simulink model "bara_thrust_model"  (R2018a)
settings: Solver=FixedStepAuto  StartTime=0.0  StopTime=sim_data3(end,1)  FixedStep=0.0104  RelTol=1e-3
PreLoadFcn:
  | a = 0.03432;
  | b = 0.3933;
  | c = 0.0056;
model workspace (MAT data in the model file):
  a = 0.00307384410727
  a1 = Simulink.Parameter
  a1.Value = 0.03432
  a1.DataType = 'double'
  a1.Dimensions = [1 1]
  b = 0.991162737935
  b1 = Simulink.Parameter
  b1.Value = 0.3933
  b1.DataType = 'auto'
  b1.Dimensions = [1 1]
  c = 0.0571408330036
  c1 = Simulink.Parameter
  c1.Value = 0.0056
  c1.DataType = 'auto'
  c1.Dimensions = [1 1]
  d = 1.70754777062
  e = 2.1214749593
settings Model: ParameterArgumentNames=a,a1,b,b1,c,c1  OrderedModelArguments=off  Creator=emran  LastModifiedBy=emran

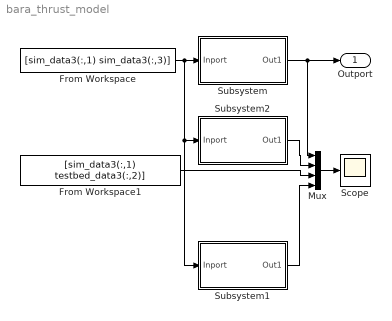
== system bara_thrust_model ==
  From Workspace : FromWorkspace  VariableName=[sim_data3(:,1) sim_data3(:,3)]  SampleTime=0
  From Workspace1 : FromWorkspace  VariableName=[sim_data3(:,1) testbed_data3(:,2)]  SampleTime=0
  Mux : Mux
  Scope : Scope
  Subsystem : Subsystem
  Subsystem1 : Subsystem
  Subsystem2 : Subsystem
  Outport : Outport
  wires:
  From Workspace/1 -> Subsystem2/1(Inport), Subsystem1/1(Inport), Subsystem/1(Inport)
  Subsystem/1(Out1) -> Mux/1, Outport/1
  From Workspace1/1 -> Mux/3
  Mux/1 -> Scope/1
  Subsystem1/1(Out1) -> Mux/4
  Subsystem2/1(Out1) -> Mux/2

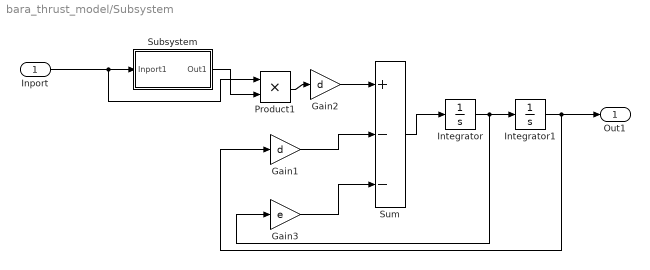
== system bara_thrust_model/Subsystem ==
  Inport : Inport
  Gain1 : Gain  Gain=d
  Gain2 : Gain  Gain=d
  Gain3 : Gain  Gain=e
  Integrator : Integrator
  Integrator1 : Integrator
  Product1 : Product
  Subsystem : Subsystem
  Sum : Sum  Inputs=+--
  Out1 : Outport
  wires:
  Subsystem/1(Out1) -> Product1/2
  Inport/1 -> Product1/1, Subsystem/1(Inport1)
  Integrator/1 -> Gain3/1, Integrator1/1
  Product1/1 -> Gain2/1
  Gain2/1 -> Sum/1
  Integrator1/1 -> Out1/1, Gain1/1
  Sum/1 -> Integrator/1
  Gain3/1 -> Sum/3
  Gain1/1 -> Sum/2

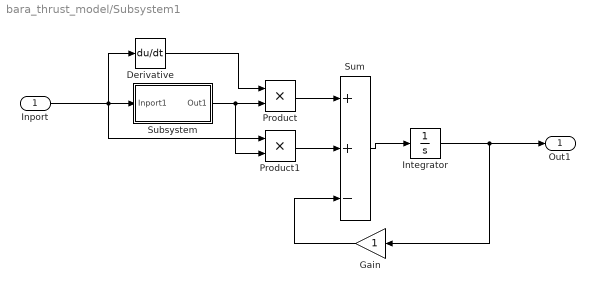
== system bara_thrust_model/Subsystem1 ==
  Inport : Inport
  Derivative : Derivative
  Gain : Gain
  Integrator : Integrator
  Product : Product
  Product1 : Product
  Subsystem : Subsystem
  Sum : Sum  Inputs=++-
  Out1 : Outport
  wires:
  Derivative/1 -> Product/1
  Product1/1 -> Sum/2
  Inport/1 -> Subsystem/1(Inport1), Derivative/1, Product1/1
  Integrator/1 -> Out1/1, Gain/1
  Subsystem/1(Out1) -> Product/2, Product1/2
  Sum/1 -> Integrator/1
  Product/1 -> Sum/1
  Gain/1 -> Sum/3

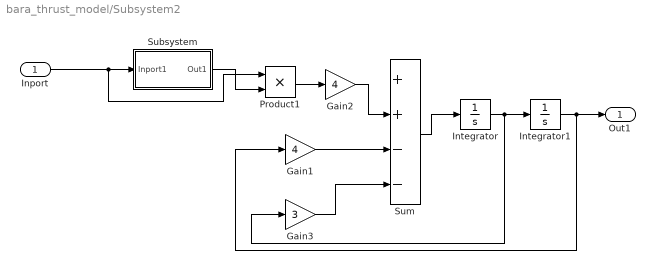
== system bara_thrust_model/Subsystem2 ==
  Inport : Inport
  Gain1 : Gain  Gain=4
  Gain2 : Gain  Gain=4
  Gain3 : Gain  Gain=3
  Integrator : Integrator
  Integrator1 : Integrator
  Product1 : Product
  Subsystem : Subsystem
  Sum : Sum  Inputs=++--
  Out1 : Outport
  wires:
  Subsystem/1(Out1) -> Product1/2
  Inport/1 -> Product1/1, Subsystem/1(Inport1)
  Product1/1 -> Gain2/1
  Sum/1 -> Integrator/1
  Integrator/1 -> Gain3/1, Integrator1/1
  Gain1/1 -> Sum/3
  Gain3/1 -> Sum/4
  Integrator1/1 -> Gain1/1, Out1/1
  Gain2/1 -> Sum/2

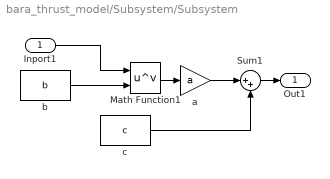
== system bara_thrust_model/Subsystem/Subsystem ==
  Inport1 : Inport
  Math Function1 : Math  Operator=pow  SaturateOnIntegerOverflow=on
  Sum1 : Sum  Inputs=|++
  a : Gain  Gain=a
  b : Constant  Value=b
  c : Constant  Value=c
  Out1 : Outport
  wires:
  c/1 -> Sum1/2
  Sum1/1 -> Out1/1
  Math Function1/1 -> a/1
  Inport1/1 -> Math Function1/1
  a/1 -> Sum1/1
  b/1 -> Math Function1/2

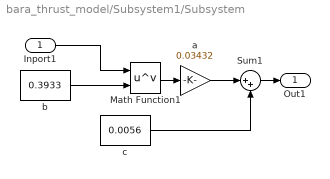
== system bara_thrust_model/Subsystem1/Subsystem ==
  Inport1 : Inport
  Math Function1 : Math  Operator=pow  SaturateOnIntegerOverflow=on
  Sum1 : Sum  Inputs=|++
  a : Gain  Gain=0.03432
  b : Constant  Value=0.3933
  c : Constant  Value=0.0056
  Out1 : Outport
  wires:
  b/1 -> Math Function1/2
  a/1 -> Sum1/1
  Inport1/1 -> Math Function1/1
  Math Function1/1 -> a/1
  Sum1/1 -> Out1/1
  c/1 -> Sum1/2

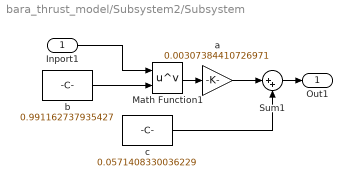
== system bara_thrust_model/Subsystem2/Subsystem ==
  Inport1 : Inport
  Math Function1 : Math  Operator=pow  SaturateOnIntegerOverflow=on
  Sum1 : Sum  Inputs=|++
  a : Gain  Gain=0.00307384410726971
  b : Constant  Value=0.991162737935427
  c : Constant  Value=0.0571408330036229
  Out1 : Outport
  wires:
  c/1 -> Sum1/2
  Sum1/1 -> Out1/1
  Math Function1/1 -> a/1
  Inport1/1 -> Math Function1/1
  a/1 -> Sum1/1
  b/1 -> Math Function1/2
